simulink model "test_joystick"  (R2022a)
settings: Solver=VariableStepAuto  StartTime=0.0  StopTime=inf  RelTol=1e-3
libraries: vrlib x1
settings Model: SimulationMode=accelerator  Creator=김응태  LastModifiedBy=USer

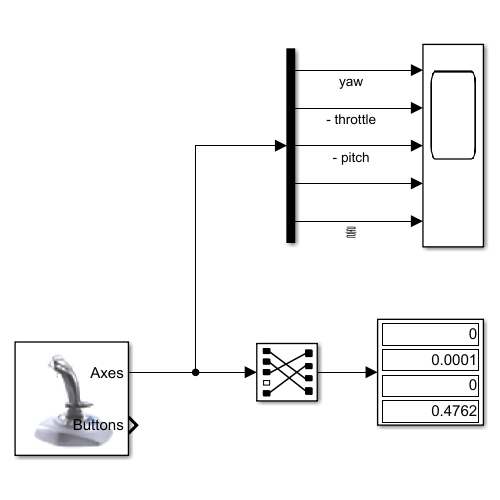
[thumbnail: Simulink's stored preview of the top-level diagram]
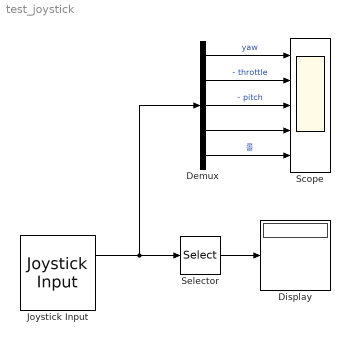
== system test_joystick ==
  Demux : Demux  Outputs=5
  Display : Display
  Joystick Input : vrlib/Joystick Input  joyid=1  adjustports=on  forcefeed=off
  Scope : Scope  NumInputPorts=5
  Selector : Selector  InputPortWidth=5  IndexOptions=Index vector (dialog)  Indices="[3 5  1 2]"  OutputSizes=1
  wires:
  Joystick Input/1 -> Demux/1, Selector/1
  Demux/1 -> Scope/1  "yaw"
  Demux/2 -> Scope/2  "- throttle"
  Demux/3 -> Scope/3  "- pitch"
  Demux/4 -> Scope/4
  Demux/5 -> Scope/5  "롤"
  Selector/1 -> Display/1
